simulink model "xiankong03_nolinearv3"  (Simulink 9.0)
settings: Solver=VariableStepAuto  StartTime=0.0  StopTime=10.0  RelTol=1e-3
values from neighbouring files (symbols this model uses):
  A = [1 0;0 2]    [xiankong01.m]    (also in xiankong02.m; xiankong03.m; xiankong03v2.m; xiankong03v4.m)
  B = [1;1]    [xiankong01.m]    (also in xiankong02.m; xiankong03.m; xiankong03v2.m; xiankong03v4.m)
  C = -C    [xiankong01.m]    (also in xiankong02.m; xiankong03.m = [1 2]; xiankong03v2.m = [1 2]; xiankong03v4.m = [1 2])
  K1 = K(1:2)    [xiankong03.m]    (also in xiankong03v2.m; xiankong03v4.m; xiankong04.m; xiankong04v2.m)
  K2 = K(3)    [xiankong03.m]    (also in xiankong03v2.m; xiankong03v4.m; xiankong04.m; xiankong04v2.m)
libraries: simulink x1
settings Model: Creator=wulin  LastModifiedBy=wulin
settings DataIOCC: SaveFormat=Dataset
settings OptimizationCC: LifeSpan=auto
settings DebuggingCC: UnderspecifiedInitializationDetection=Simplified  MergeDetectMultiDrivingBlocksExec=error  SFUnexpectedBacktrackingDiag=error  SFNoUnconditionalDefaultTransitionDiag=error  SFExecutionAtInitializationDiag=warning
settings HardwareCC: ProdBitPerPointer=64  ProdBitPerSizeT=64  ProdBitPerPtrDiffT=64  ProdLargestAtomicFloat=Float  ProdIntDivRoundTo=Zero  ProdEndianess=LittleEndian  ProdWordSize=64  ProdHWDeviceType=Intel->x86-64 (Windows64)
settings ModelReferenceCC: PropagateSignalLabelsOutOfModel=on
settings CodeAppCC: StateflowObjectComments=off
settings GRTTargetCC: TargetLangStandard=C99 (ISO)
settings ConfigComp: CovMetricSettings=dwe  CovHtmlReporting=off  CovSaveCumulativeToWorkspaceVar=off  CovSaveSingleToWorkspaceVar=off  CovExternalEMLEnable=on

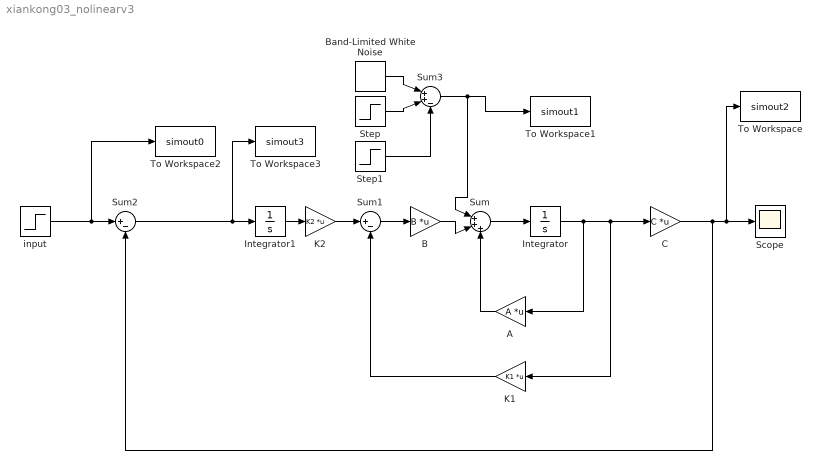
== system xiankong03_nolinearv3 ==
  "A " : Gain  Gain=A  Multiplication=Matrix(K*u) (u vector)
  B : Gain  Gain=B  Multiplication=Matrix(K*u) (u vector)
  Band-Limited White Noise : simulink/Sources/Band-Limited White Noise  Cov=0.01  Ts=0.01  seed=[23341]
  C : Gain  Gain=C  Multiplication=Matrix(K*u) (u vector)
  Integrator : Integrator
  Integrator1 : Integrator
  "K1 " : Gain  Gain=K1  Multiplication=Matrix(K*u) (u vector)
  K2 : Gain  Gain=K2  Multiplication=Matrix(K*u) (u vector)
  Scope : Scope
  Step : Step  SampleTime=0
  Step1 : Step  Time=2  SampleTime=0
  Sum : Sum  Inputs=|+++
  Sum1 : Sum  Inputs=|+-
  Sum2 : Sum  Inputs=|+-
  Sum3 : Sum  Inputs=|++-
  To Workspace : ToWorkspace  VariableName=simout2  SampleTime=-1
  To Workspace1 : ToWorkspace  VariableName=simout1  SampleTime=-1
  To Workspace2 : ToWorkspace  VariableName=simout0  SampleTime=-1
  To Workspace3 : ToWorkspace  VariableName=simout3  SampleTime=-1
  input : Step  SampleTime=0
  wires:
  Integrator/1 -> C/1, "K1 "/1, "A "/1
  C/1 -> Sum2/2, To Workspace/1, Scope/1
  "K1 "/1 -> Sum1/2
  Sum/1 -> Integrator/1
  Integrator1/1 -> K2/1
  K2/1 -> Sum1/1
  Sum1/1 -> B/1
  input/1 -> Sum2/1, To Workspace2/1
  "A "/1 -> Sum/3
  B/1 -> Sum/2
  Band-Limited White Noise/1 -> Sum3/1
  Step/1 -> Sum3/2
  Step1/1 -> Sum3/3
  Sum3/1 -> Sum/1, To Workspace1/1
  Sum2/1 -> Integrator1/1, To Workspace3/1
